simulink model "motomatic_pendGA"  (R2021a)
settings: Solver=ode15s  StartTime=0.0  StopTime=10.0  FixedStep=1*10^-5  RelTol=1e-5
values from neighbouring files (symbols this model uses):
  Ka = 5.1793    [TestGA.m]    (also in TestGAold.m; simFunctGAMod.m)
  Kp = 4.90379    [TestGA.m]    (also in TestGAold.m; simFunctGAMod.m)
  Kt = .1429    (= 0.1429)    [TestGA.m]    (also in TestGAold.m; simFunctGAMod.m)
  N = 8.1    [TestGA.m]    (also in TestGAold.m; simFunctGAMod.m)
  physParam = [m, L, g, vmo, N]    [TestGA.m]    (also in TestGAold.m)
  th_init = deg2rad(110)    [TestGA.m]    (also in TestGAold.m)
settings Model: Creator=Bradley Kwan  LastModifiedBy=MikeyG
settings SolverCC: AlgebraicLoopSolver=TrustRegion
settings DataIOCC: SaveFormat=Array
settings DebuggingCC: SFMachineParentedDataDiag=warning

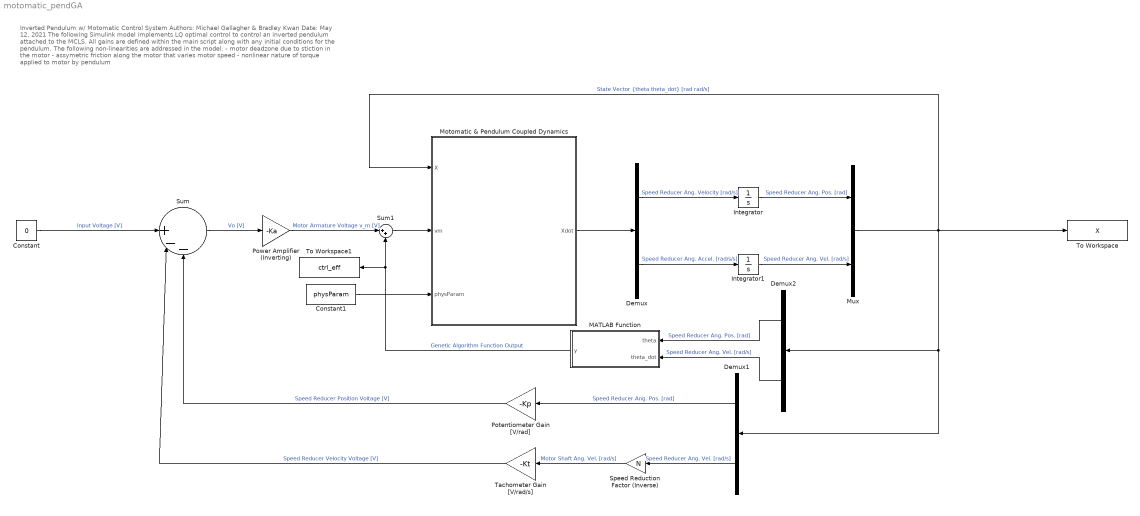
== system motomatic_pendGA ==
  note: Inverted Pendulum w/ Motomatic Control System
      | Authors: Michael Gallagher & Bradley Kwan
      | Date: May 12, 2021
      |
      | The following Simulink model implements LQ optimal control to control an inverted pendulum attached to the MCLS. All gains are defined within the main script along with any initial conditions for the pendulum. The following non-linearities are addressed in the model:
      |
      | - motor deadzone due to stiction in the motor
      | - assymetric friction along the motor that varies motor speed
      | - nonlinear nature of torque applied to motor by pendulum
  Constant : Constant  Value=0
  Constant1 : Constant  Value=physParam
  Demux : Demux  Outputs=2
  Demux1 : Demux  Outputs=2
  Demux2 : Demux  Outputs=2
  Integrator : Integrator  InitialCondition=th_init
  Integrator1 : Integrator
  MATLAB Function : MATLAB Function  TreatAsAtomicUnit=on
  Motomatic & Pendulum Coupled Dynamics : MATLAB Function  TreatAsAtomicUnit=on
  Mux : Mux  Inputs=2
  Potentiometer Gain [V/rad] : Gain  Gain=-Kp
  Power Amplifier (Inverting) : Gain  Gain=-Ka
  Speed Reduction Factor (Inverse) : Gain  Gain=N
  Sum : Sum  Inputs=||+--
  Sum1 : Sum  Inputs=|++
  Tachometer Gain [V/rad/s] : Gain  Gain=-Kt
  To Workspace : ToWorkspace  VariableName=X  SampleTime=-1
  To Workspace1 : ToWorkspace  VariableName=ctrl_eff  SampleTime=-1
  wires:
  Sum/1 -> Power Amplifier (Inverting)/1  "Vo [V]"
  Constant/1 -> Sum/1  "Input Voltage [V]"
  Constant1/1 -> Motomatic & Pendulum Coupled Dynamics/3(physParam)
  Motomatic & Pendulum Coupled Dynamics/1(Xdot) -> Demux/1
  Demux/1 -> Integrator/1  "Speed Reducer Ang. Velocity [rad/s]"
  Demux/2 -> Integrator1/1  "Speed Reducer Ang. Accel. [rad/s/s]"
  Integrator/1 -> Mux/1  "Speed Reducer Ang. Pos. [rad]"
  Integrator1/1 -> Mux/2  "Speed Reducer Ang. Vel. [rad/s]"
  Mux/1 -> To Workspace/1, Motomatic & Pendulum Coupled Dynamics/1(X), Demux2/1, Demux1/1  "State Vector {theta theta_dot} [rad rad/s]"
  Demux1/2 -> Speed Reduction Factor (Inverse)/1  "Speed Reducer Ang. Vel. [rad/s]"
  Demux1/1 -> Potentiometer Gain [V/rad]/1  "Speed Reducer Ang. Pos. [rad]"
  Speed Reduction Factor (Inverse)/1 -> Tachometer Gain [V/rad/s]/1  "Motor Shaft Ang. Vel. [rad/s]"
  Potentiometer Gain [V/rad]/1 -> Sum/3  "Speed Reducer Position Voltage [V]"
  MATLAB Function/1(y) -> Sum1/2, To Workspace1/1  "Genetic Algorithm Function Output"
  Power Amplifier (Inverting)/1 -> Sum1/1  "Motor Armature Voltage v_m [V]"
  Sum1/1 -> Motomatic & Pendulum Coupled Dynamics/2(vm)
  Tachometer Gain [V/rad/s]/1 -> Sum/2  "Speed Reducer Velocity Voltage [V]"
  Demux2/1 -> MATLAB Function/1(theta)  "Speed Reducer Ang. Pos. [rad]"
  Demux2/2 -> MATLAB Function/2(theta_dot)  "Speed Reducer Ang. Vel. [rad/s]"

== matlab function motomatic_pendGA/Motomatic & Pendulum Coupled Dynamics ==
  data: X input; Xdot output; vm input; physParam input
function Xdot = motor_dynamics(X,vm, physParam)

% First define the physical parameters of the pendulum model
M = physParam(1);      % bob mass [kg]
L = physParam(2);      % pendulum length [m]
g = physParam(3);      % gravitational acceleration [m/s/s]
vmo = physParam(4);    % Voltage necessary to hold pendulum at 90 degrees [v]
N = physParam(5);      % speed reducer factor

% Based on the physical parameters of the model, find the polar moments of
% inertia of the motor and pendulum
J_p = M*L^2;                    % Polar moment inertia of pendulum [kg*m^2]
J_m = M*g*L/vmo*(.2740/19.763); % Polar moment inertia of motor [kg*m^2]

Xdot = [NaN NaN];

% First the function tests to see if the motor will overcome stiction
if abs(vm) < .8316 && X(2) == 0 
    Xdot = [0 0];
else
    % Assymetric friction function to determine tau_m F(x(1))
    % tau_m = .274;    % using the linearized time constant for now...
    tau_m = polyval(X(1) + pi,[0.000692604307959516,-0.0237914958272148,0.353136055910927,-2.96560343582695,15.4980953250600,-52.2330200420004,113.848925236937,-156.621218542920,128.406743766801,-55.8405504744871,9.90619154457846]);
    tau_m = tau_m(1);
    Xdot(1) = X(2);
    Xdot(2) = -N*J_m/tau_m/(N*J_m+J_p)*X(2) ...
              +M*g*L*sin(X(1))/(N*J_m+J_p) + ...
              M*g*L/(vmo*(N*J_m+J_p))*vm;
end

== matlab function motomatic_pendGA/MATLAB Function ==
  data: theta input; y output; theta_dot input
function y = fcn(theta, theta_dot)

y = simFunctGA(theta, theta_dot);
